simulink model "nn_blackbox"  (R2020b)
settings: Solver=VariableStepAuto  StartTime=0.0  StopTime=1  RelTol=1e-3
values from neighbouring files (symbols this model uses):
  b_1 = 2.14    [nn_sample.mat]
  b_2 = 1.29    [nn_sample.mat]
  b_3 = -0.58    [nn_sample.mat]
  w_1 = -34.4    [nn_sample.mat]
  w_2 = -2.52    [nn_sample.mat]
  w_3 = -1.3    [nn_sample.mat]
  w_4 = 2.28    [nn_sample.mat]
libraries: neural x2
settings Model: Creator=RodolfoSalvador  LastModifiedBy=RodolfoSalvador

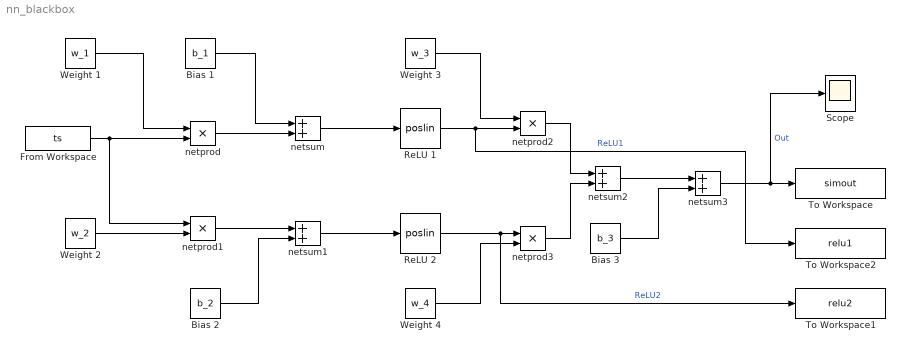
== system nn_blackbox ==
  Bias 1 : Constant  Value=b_1
  Bias 2 : Constant  Value=b_2
  Bias 3 : Constant  Value=b_3
  From Workspace : FromWorkspace  VariableName=ts  SampleTime=1e-3
  ReLU 1 : neural/Transfer Functions/poslin
      settings: SourceProductBaseCode=NN
  ReLU 2 : neural/Transfer Functions/poslin
      settings: SourceProductBaseCode=NN
  Scope : Scope
  To Workspace : ToWorkspace  VariableName=simout  SampleTime=-1
  To Workspace1 : ToWorkspace  VariableName=relu2  SampleTime=-1
  To Workspace2 : ToWorkspace  VariableName=relu1  SampleTime=-1
  Weight 1 : Constant  Value=w_1
  Weight 2 : Constant  Value=w_2
  Weight 3 : Constant  Value=w_3
  Weight 4 : Constant  Value=w_4
  netprod{,1..3} (4 alike) : Product  InputSameDT=on  RndMeth=Zero  SaturateOnIntegerOverflow=on  OutDataTypeStr=Inherit: Same as first input
  netsum{,1..3} (4 alike) : Sum  Inputs=2  InputSameDT=on  SaturateOnIntegerOverflow=on  OutDataTypeStr=Inherit: Same as first input
  wires:
  From Workspace/1 -> netprod1/1, netprod/2
  Weight 1/1 -> netprod/1
  netprod/1 -> netsum/2
  Bias 1/1 -> netsum/1
  Weight 2/1 -> netprod1/2
  netprod1/1 -> netsum1/1
  Bias 2/1 -> netsum1/2
  netsum/1 -> ReLU 1/1
  netsum1/1 -> ReLU 2/1
  ReLU 1/1 -> To Workspace2/1, netprod2/2  "ReLU1"
  Weight 3/1 -> netprod2/1
  ReLU 2/1 -> To Workspace1/1, netprod3/1  "ReLU2"
  Weight 4/1 -> netprod3/2
  netprod2/1 -> netsum2/1
  netprod3/1 -> netsum2/2
  netsum2/1 -> netsum3/1
  Bias 3/1 -> netsum3/2
  netsum3/1 -> Scope/1, To Workspace/1  "Out"
